simulink model "Prob6"  (R2020b)
settings: Solver=VariableStepAuto  StartTime=0.0  StopTime=100  RelTol=1e-3
settings Model: Creator=stkaravind  LastModifiedBy=stkaravind

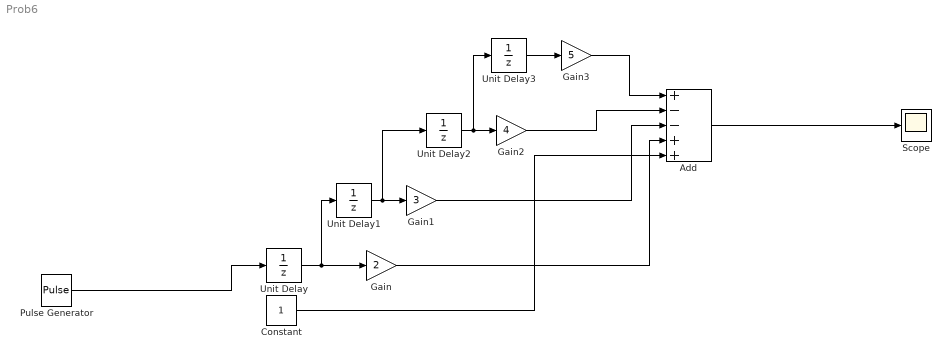
== system Prob6 ==
  Add : Sum  Inputs=+--++
  Constant : Constant
  Gain : Gain  Gain=2
  Gain1 : Gain  Gain=3
  Gain2 : Gain  Gain=4
  Gain3 : Gain  Gain=5
  Pulse Generator : DiscretePulseGenerator  PulseType=Time based  Period=10  PulseWidth=5
  Scope : Scope
  Unit Delay{,1..3} (4 alike) : UnitDelay  SampleTime=-1  HasFrameUpgradeWarning=on
  wires:
  Unit Delay/1 -> Gain/1, Unit Delay1/1
  Gain3/1 -> Add/1
  Add/1 -> Scope/1
  Unit Delay3/1 -> Gain3/1
  Gain1/1 -> Add/3
  Gain2/1 -> Add/2
  Unit Delay2/1 -> Gain2/1, Unit Delay3/1
  Unit Delay1/1 -> Gain1/1, Unit Delay2/1
  Gain/1 -> Add/4
  Constant/1 -> Add/5
  Pulse Generator/1 -> Unit Delay/1
